simulink model "Convertidores_grados"  (R2023a)
settings: Solver=VariableStepAuto  StartTime=0.0  StopTime=10.0  RelTol=1e-3
undefined symbols (not defined in the file or in its folder): T
settings Model: Creator=Nacho Andrade  LastModifiedBy=Nacho Andrade

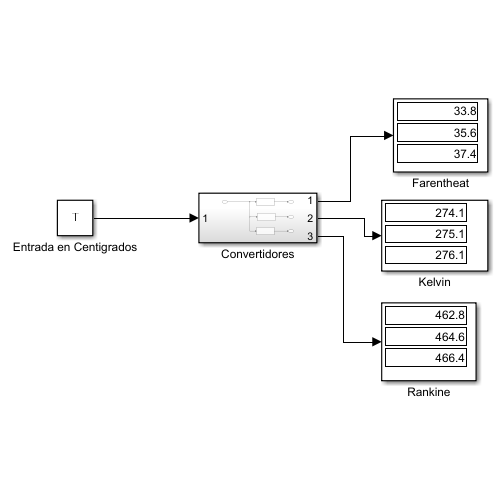
[thumbnail: Simulink's stored preview of the top-level diagram]
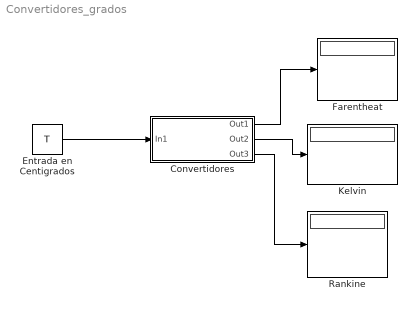
== system Convertidores_grados ==
  Convertidores : Subsystem
  Entrada en Centigrados : Constant  Value=T
  Farentheat : Display
  Kelvin : Display
  Rankine : Display
  wires:
  Convertidores/1(Out1) -> Farentheat/1
  Convertidores/2(Out2) -> Kelvin/1
  Convertidores/3(Out3) -> Rankine/1
  Entrada en Centigrados/1 -> Convertidores/1(In1)

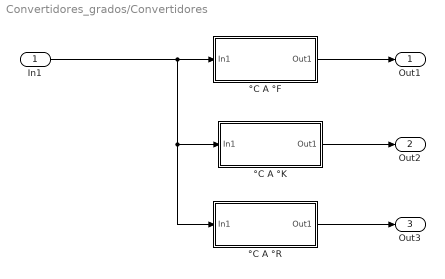
== system Convertidores_grados/Convertidores ==
  In1 : Inport
  °C A °F : Subsystem
  °C A °K : Subsystem
  °C A °R : Subsystem
  Out1 : Outport
  Out2 : Outport  Port=2
  Out3 : Outport  Port=3
  wires:
  °C A °K/1(Out1) -> Out2/1
  °C A °F/1(Out1) -> Out1/1
  In1/1 -> °C A °R/1(In1), °C A °K/1(In1), °C A °F/1(In1)
  °C A °R/1(Out1) -> Out3/1

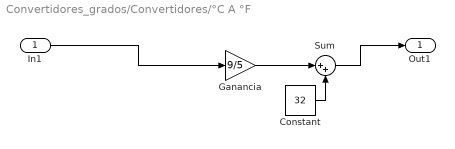
== system Convertidores_grados/Convertidores/°C A °F ==
  In1 : Inport
  Constant : Constant  Value=32
  Ganancia : Gain  Gain=9/5
  Sum : Sum  Inputs=|++
  Out1 : Outport
  wires:
  Constant/1 -> Sum/2
  In1/1 -> Ganancia/1
  Sum/1 -> Out1/1
  Ganancia/1 -> Sum/1

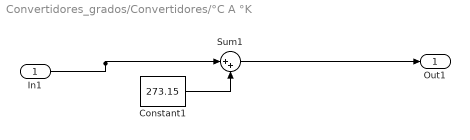
== system Convertidores_grados/Convertidores/°C A °K ==
  In1 : Inport
  Constant1 : Constant  Value=273.15
  Sum1 : Sum  Inputs=|++
  Out1 : Outport
  wires:
  Sum1/1 -> Out1/1
  In1/1 -> Sum1/1
  Constant1/1 -> Sum1/2

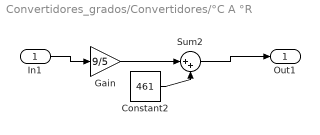
== system Convertidores_grados/Convertidores/°C A °R ==
  In1 : Inport
  Constant2 : Constant  Value=461
  Gain : Gain  Gain=9/5
  Sum2 : Sum  Inputs=|++
  Out1 : Outport
  wires:
  Gain/1 -> Sum2/1
  In1/1 -> Gain/1
  Constant2/1 -> Sum2/2
  Sum2/1 -> Out1/1
